simulink model "pendulum"  (R2021b)
settings: Solver=ode45  StartTime=0.0  StopTime=80  RelTol=1e-3
values from neighbouring files (symbols this model uses):
  c = [1 0]'    [lab2.m]    (also in var.m = 0.00035)
  d = [0 0]'    [lab2.m]    (also in var.m = 0.023)
  g = 9.8    [var.m]
  J = .009    (= 0.009)    [var.m]
  L = .495    (= 0.495)    [var.m]
  m = .43    (= 0.43)    [var.m]
libraries: simulink_extras x2, fuzblock x1
settings Model: Creator=nbelo  LastModifiedBy=nbelo
settings SolverCC: ZeroCrossControl=DisableAll
settings OptimizationCC: BooleanDataType=off

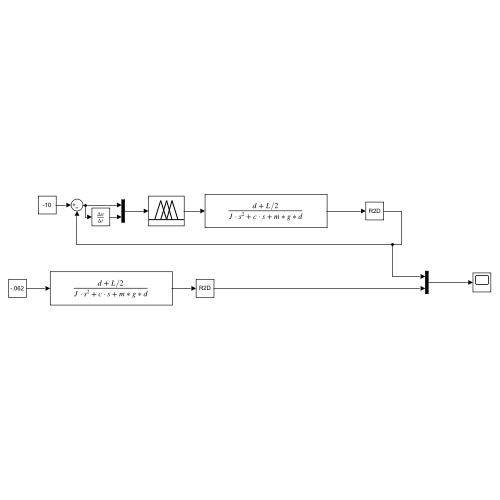
[thumbnail: Simulink's stored preview of the top-level diagram]
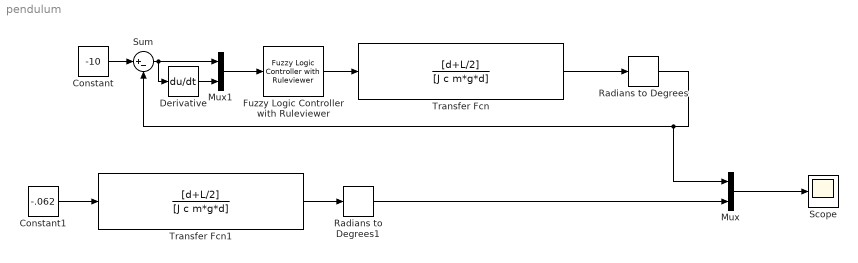
== system pendulum ==
  Constant : Constant  Value=-10
  Constant1 : Constant  Value=-.062
  Derivative : Derivative
  Fuzzy Logic Controller with Ruleviewer : fuzblock/Fuzzy Logic  Controller  with Ruleviewer  fismatrix=fuzzyCon  Ts=2
  Mux : Mux  Inputs=2
  Mux1 : Mux  Inputs=2
  Radians to Degrees : simulink_extras/Transformations/Radians to Degrees
  Radians to Degrees1 : simulink_extras/Transformations/Radians to Degrees
  Scope : Scope
  Sum : Sum  Inputs=|+-
  Transfer Fcn : TransferFcn  Numerator=[d+L/2]  Denominator=[J c m*g*d]
  Transfer Fcn1 : TransferFcn  Numerator=[d+L/2]  Denominator=[J c m*g*d]
  wires:
  Transfer Fcn1/1 -> Radians to Degrees1/1
  Radians to Degrees1/1 -> Mux/2
  Radians to Degrees/1 -> Mux/1, Sum/2
  Transfer Fcn/1 -> Radians to Degrees/1
  Fuzzy Logic Controller with Ruleviewer/1 -> Transfer Fcn/1
  Mux1/1 -> Fuzzy Logic Controller with Ruleviewer/1
  Constant/1 -> Sum/1
  Sum/1 -> Derivative/1, Mux1/1
  Derivative/1 -> Mux1/2
  Constant1/1 -> Transfer Fcn1/1
  Mux/1 -> Scope/1
